simulink model "motiongen_pos"  (R2021a)
settings: Solver=FixedStepDiscrete  StartTime=0.0  StopTime=10.0  FixedStep=0.01  RelTol=1e-3  EnableMultiTasking=on
settings Model: Creator=ihout_000  LastModifiedBy=ihout
settings SolverCC: AlgebraicLoopSolver=TrustRegion
settings DataIOCC: LimitDataPoints=on  SaveFormat=Array
settings OptimizationCC: ExpressionDepthLimit=2147483647  LifeSpan=inf  SimCompilerOptimization=on
settings DebuggingCC: SolverPrmCheckMsg=warning  StateNameClashWarn=warning  SFUnexpectedBacktrackingDiag=warning  SFNoUnconditionalDefaultTransitionDiag=warning  SFExecutionAtInitializationDiag=none  ArithmeticOperatorsInVariantConditions=warning
settings ModelReferenceCC: UpdateModelReferenceTargets=Force  PropagateSignalLabelsOutOfModel=off
settings SFSimCC: SimUserIncludeDirs=ruckig\include\  SimUserDefines=_USE_MATH_DEFINES  SimUseLocalCustomCode=off  CustomCodeUndefinedFunction=UseInterfaceOnly  SimTargetLang=C++
settings SFSimCC: SimUserSources=|
  | ruckig/src/ruckig/brake.cpp
  | ruckig/src/ruckig/position_first_step1.cpp
  | ruckig/src/ruckig/position_first_step2.cpp
  | ruckig/src/ruckig/position_second_step1.cpp
  | ruckig/src/ruckig/position_second_step2.cpp
  | ruckig/src/ruckig/position_third_step1.cpp
  | ruckig/src/ruckig/position_third_step2.cpp
  | ruckig/src/ruckig/velocity_second_step1.cpp
  | ruckig/src/ruckig/velocity_second_step2.cpp
  | ruckig/src/ruckig/velocity_third_step1.cpp
  | ruckig/src/ruckig/velocity_third_step2.cpp
settings RTWCC: RTWUseLocalCustomCode=off  CustomInclude=ruckig\include\  CustomDefine=_USE_MATH_DEFINES  Toolchain=Microsoft Visual C++ 2019 v16.0 | nmake (64-bit Windows)  BuildConfiguration=Specify  TargetLang=C++  RTWCustomCompilerOptimizations=/std:c++17  DLArmComputeVersion=20.02.1
settings RTWCC: CustomSource=|
  | ruckig/src/ruckig/brake.cpp
  | ruckig/src/ruckig/position_first_step1.cpp
  | ruckig/src/ruckig/position_first_step2.cpp
  | ruckig/src/ruckig/position_second_step1.cpp
  | ruckig/src/ruckig/position_second_step2.cpp
  | ruckig/src/ruckig/position_third_step1.cpp
  | ruckig/src/ruckig/position_third_step2.cpp
  | ruckig/src/ruckig/velocity_second_step1.cpp
  | ruckig/src/ruckig/velocity_second_step2.cpp
  | ruckig/src/ruckig/velocity_third_step1.cpp
  | ruckig/src/ruckig/velocity_third_step2.cpp
settings CodeAppCC: StateflowObjectComments=on
settings GRTTargetCC: TargetLangStandard=C++03 (ISO)
settings ConfigComp: CovMetricSettings=dw  CovSaveCumulativeToWorkspaceVar=on  CovSaveSingleToWorkspaceVar=on  CovExternalEMLEnable=off  CovBoundaryAbsTol=1.0e-5

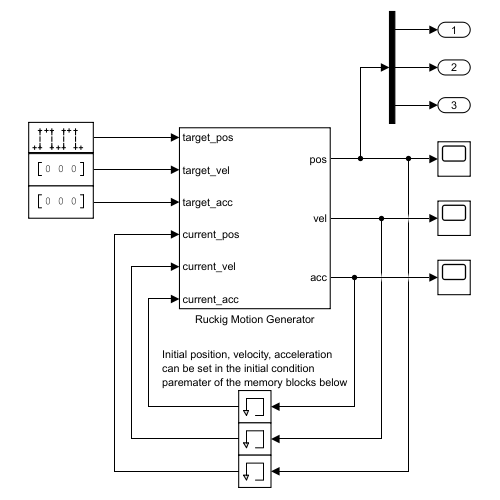
[thumbnail: Simulink's stored preview of the top-level diagram]
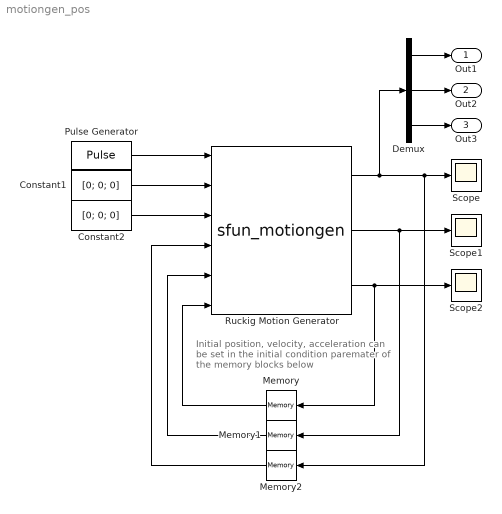
== system motiongen_pos ==
  note: Initial position, velocity, acceleration
      | can be set in the initial condition
      | paremater of the memory blocks below
  Constant1 : Constant  Value=[0; 0; 0]
  Constant2 : Constant  Value=[0; 0; 0]
  Demux : Demux  Outputs=3
  Memory : Memory  InitialCondition=[0 0 0]  InheritSampleTime=on
  Memory1 : Memory  InitialCondition=[0 0 0]  InheritSampleTime=on
  Memory2 : Memory  InitialCondition=[2 -1 1]  InheritSampleTime=on
  Pulse Generator : DiscretePulseGenerator  Amplitude=[10; 1; 5]  Period=500  PulseWidth=200  SampleTime=0.01
  Ruckig Motion Generator : S-Function  FunctionName=sfun_motiongen  Parameters=ts,ndofs,vmax,amax,jmax,control,sync,duration  SFunctionDeploymentMode=off  EnableBusSupport=off  mask{ts=1e-2, ndofs=3, vmax=[15 10 25], amax=[150 100 50], jmax=[500 1000 700], sync=TIME_SYNCHRONIZATION_IF_NECESSARY, duration=DISCRETE, control=POSITION}
      mask prompts: ts "Sample Time:"; ndofs "Number of DoF's:"; vmax "Maximum Velocity Vector:"; amax "Maximum Acceleration Vector:"; jmax "Maximum Jerk Vector:"; sync "Synchronization Behavior:"; duration "Duration Discretization:"; control "Control Interface:"
      mask TypeOptions sync: NO_SYNCHRONIZATION | TIME_SYNCHRONIZATION_IF_NECESSARY | ONLY_TIME_SYNCHRONIZATION | ONLY_PHASE_SYNCHRONIZATION
      mask TypeOptions duration: CONTINUOUS | DISCRETE
      mask TypeOptions control: POSITION | VELOCITY
      mask Display:
      | port_label('input', 1, 'target_pos')
      | port_label('input', 2, 'target_vel')
      | port_label('input', 3, 'target_acc')
      | port_label('input', 4, 'current_pos')
      | port_label('input', 5, 'current_vel')
      | port_label('input', 6, 'current_acc')
      | port_label('output', 1, 'pos')
      | port_label('output', 2, 'vel')
      | port_label('output', 3, 'acc')
  Scope : Scope
  Scope1 : Scope
  Scope2 : Scope
  Out1 : Outport  VectorParamsAs1DForOutWhenUnconnected=off
  Out2 : Outport  Port=2  VectorParamsAs1DForOutWhenUnconnected=off
  Out3 : Outport  Port=3  VectorParamsAs1DForOutWhenUnconnected=off
  wires:
  Pulse Generator/1 -> Ruckig Motion Generator/1
  Constant1/1 -> Ruckig Motion Generator/2
  Ruckig Motion Generator/1 -> Demux/1, Memory2/1, Scope/1
  Ruckig Motion Generator/2 -> Memory1/1, Scope1/1
  Ruckig Motion Generator/3 -> Memory/1, Scope2/1
  Demux/1 -> Out1/1
  Demux/2 -> Out2/1
  Demux/3 -> Out3/1
  Memory/1 -> Ruckig Motion Generator/6
  Memory1/1 -> Ruckig Motion Generator/5
  Memory2/1 -> Ruckig Motion Generator/4
  Constant2/1 -> Ruckig Motion Generator/3
